simulink model "experiment_1"  (R2019a)
settings: Solver=VariableStepAuto  StartTime=0.0  StopTime=150  RelTol=1e-3
values from neighbouring files (symbols this model uses):
  b = fun(4)    [PIDtun_AHkap.m]
  c = 0.4    [TUNE_PID.m]
  Td = fun(3)*Tu    [PIDtun_AHkap.m]
  Tf = Td / N    [TUNE_PID.m]
  Ti = fun(2)*Tu    [PIDtun_AHkap.m]
  Tt = sqrt(Ti+Td)    [TUNE_PID.m]
undefined symbols (not defined in the file or in its folder): b_1, c_1, Kp, plant_1, Td_1, Tf_1, Ti_1, Tt_1
settings Model: Creator=user1  LastModifiedBy=user1

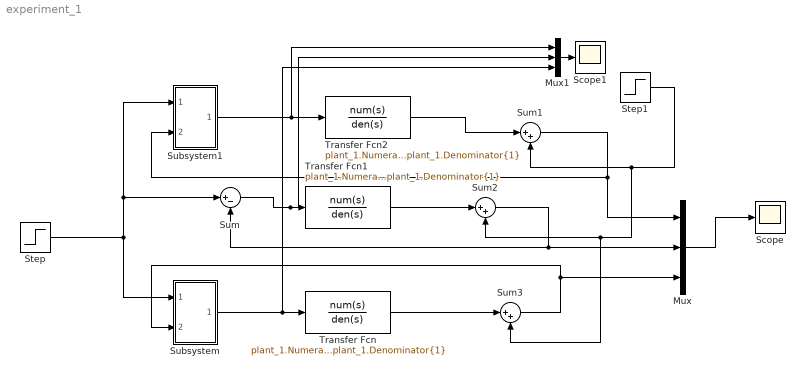
== system experiment_1 ==
  Mux : Mux  Inputs=3
  Mux1 : Mux  Inputs=3
  Scope : Scope
  Scope1 : Scope
  Step : Step  SampleTime=0
  Step1 : Step  Time=80  SampleTime=0
  Subsystem : Subsystem
  Subsystem1 : Subsystem
  Sum : Sum  Inputs=|+-
  Sum1 : Sum  Inputs=|++
  Sum2 : Sum  Inputs=|++
  Sum3 : Sum  Inputs=|++
  Transfer Fcn : TransferFcn  Numerator=plant_1.Numerator{1}  Denominator=plant_1.Denominator{1}
  Transfer Fcn1 : TransferFcn  Numerator=plant_1.Numerator{1}  Denominator=plant_1.Denominator{1}
  Transfer Fcn2 : TransferFcn  Numerator=plant_1.Numerator{1}  Denominator=plant_1.Denominator{1}
  wires:
  Step/1 -> Subsystem1/1(In1), Sum/1, Subsystem/1(In1)
  Subsystem/1(Out1) -> Mux1/3, Transfer Fcn/1
  Mux/1 -> Scope/1
  Sum/1 -> Mux1/2, Transfer Fcn1/1
  Subsystem1/1(Out1) -> Mux1/1, Transfer Fcn2/1
  Mux1/1 -> Scope1/1
  Step1/1 -> Sum3/2, Sum2/2, Sum1/2
  Transfer Fcn2/1 -> Sum1/1
  Sum1/1 -> Mux/1, Subsystem1/2(In2)
  Transfer Fcn/1 -> Sum3/1
  Transfer Fcn1/1 -> Sum2/1
  Sum3/1 -> Subsystem/2(In2), Mux/3
  Sum2/1 -> Mux/2, Sum/2

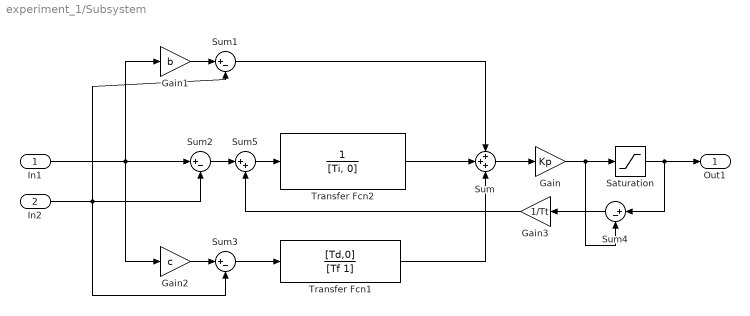
== system experiment_1/Subsystem ==
  In1 : Inport
  In2 : Inport  Port=2
  Gain : Gain  Gain=Kp
  Gain1 : Gain  Gain=b
  Gain2 : Gain  Gain=c
  Gain3 : Gain  Gain=1/Tt
  Saturation : Saturate  UpperLimit=1  LowerLimit=-1
  Sum : Sum  Inputs=+++
  Sum{1..4} (4 alike) : Sum  Inputs=|+-
  Sum5 : Sum  Inputs=|++
  Transfer Fcn1 : TransferFcn  Numerator=[Td,0]  Denominator=[Tf 1]
  Transfer Fcn2 : TransferFcn  Denominator=[Ti, 0]
  Out1 : Outport
  wires:
  Transfer Fcn1/1 -> Sum/3
  In1/1 -> Gain2/1, Sum2/1, Gain1/1
  Sum/1 -> Gain/1
  Gain2/1 -> Sum3/1
  In2/1 -> Sum2/2, Sum3/2, Sum1/2
  Sum1/1 -> Sum/1
  Sum3/1 -> Transfer Fcn1/1
  Gain1/1 -> Sum1/1
  Gain/1 -> Sum4/2, Saturation/1
  Saturation/1 -> Sum4/1, Out1/1
  Sum4/1 -> Gain3/1
  Gain3/1 -> Sum5/2
  Sum2/1 -> Sum5/1
  Sum5/1 -> Transfer Fcn2/1
  Transfer Fcn2/1 -> Sum/2

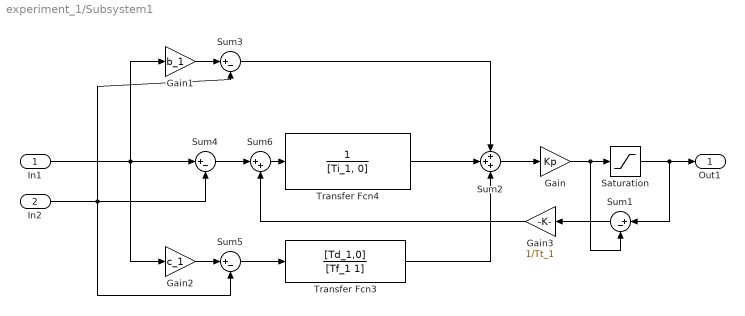
== system experiment_1/Subsystem1 ==
  In1 : Inport
  In2 : Inport  Port=2
  Gain : Gain  Gain=Kp
  Gain1 : Gain  Gain=b_1
  Gain2 : Gain  Gain=c_1
  Gain3 : Gain  Gain=1/Tt_1
  Saturation : Saturate  UpperLimit=1  LowerLimit=-1
  Sum{1,3..5} (4 alike) : Sum  Inputs=|+-
  Sum2 : Sum  Inputs=+++
  Sum6 : Sum  Inputs=|++
  Transfer Fcn3 : TransferFcn  Numerator=[Td_1,0]  Denominator=[Tf_1 1]
  Transfer Fcn4 : TransferFcn  Denominator=[Ti_1, 0]
  Out1 : Outport
  wires:
  In2/1 -> Sum4/2, Sum5/2, Sum3/2
  Transfer Fcn3/1 -> Sum2/3
  Gain2/1 -> Sum5/1
  In1/1 -> Gain2/1, Sum4/1, Gain1/1
  Sum3/1 -> Sum2/1
  Sum2/1 -> Gain/1
  Sum5/1 -> Transfer Fcn3/1
  Gain1/1 -> Sum3/1
  Transfer Fcn4/1 -> Sum2/2
  Gain/1 -> Sum1/2, Saturation/1
  Saturation/1 -> Sum1/1, Out1/1
  Sum1/1 -> Gain3/1
  Gain3/1 -> Sum6/2
  Sum4/1 -> Sum6/1
  Sum6/1 -> Transfer Fcn4/1
